simulink library "lib_lowphy"  (R2023b)
settings: Solver=VariableStepAuto  StartTime=0.0  StopTime=10.0  RelTol=1e-3
undefined symbols (not defined in the file or in its folder): AdvDSPBChannelOutDisplay, AdvDSPBDMemDisplay, AdvDSPBInDisplay, AdvDSPBOutDisplay, dpoly, dspba, dspba_ChannelInVis, dspba_ChannelOutVis, dspba_internal_get_channel_ports, evalAionMaskParam, fft_tb_in, ifft_tb_in, latency, latencyCorrection, max_FFTStages, max_NSubcarriers, primtype, UseDontCare, value
libraries: DSPBAPrim x637, DSPBAControl x55, $bdroot x16, DSPBAModelBus x12, DSPBAUtilities x6, DSPBABase x5, DSPBAWaveformSynth x4, DspbAdvFftLibrary x3, DSPBAVectorUtil x2, DspbAdvVfftPrefix x1
(part 7 of 9)

== system lib_lowphy/iFFT_B2S/B2S/B2S_Inst/CB/Rdaddr_gen1 ==
  sampleaddr_reg : Inport
  cpin : Inport  Port=2
  rba : Inport  Port=3
  fftsize : Inport  Port=4
  Lut4 : DSPBAPrim/Lut  primtype=lut  nInputs=1  nOutputs=1  omode=Specify via dialog  otype=fixdt(0,2,0)  scale=0  rndmethod=Unbiased  factor=1  satmethod=Symmetric  shift_vec=[0 1 2 -1]  value=[0 zeros(1,8) 0 1 2 3 0]  inPortNames=[' '; ' ';]  outPortNames=[' ']  dspbaimage=dspba_prim.svg  text=fprintf('LUT');  style=Optimised  visibilities=8 + 1024  floatPrecision=float32_m23  version=20211007
  Mux : DSPBAPrim/Mux  primtype=mux  nInputs=evalAionMaskParam(gcb,'value',1)+1  nOutputs=1  omode=Inherit via internal rule  otype=sfix(16)  scale=2^-15  rndmethod=Unbiased  factor=1  satmethod=Symmetric  shift_vec=[0 1 2 -1]  value=4  inPortNames=['s '; 'd0'; 'd1'; 'd2'; 'd3'; 'd4'; 'd5'; 'd6'; 'd7'; 'd8'; 'd9';]  outPortNames=[' ']  dspbaimage=dspba_prim_tall.svg  text=fprintf('%s', primtype);  style=Optimised  visibilities=1032  version=20211007
  Mux1 : DSPBAPrim/Mux  primtype=mux  nInputs=evalAionMaskParam(gcb,'value',1)+1  nOutputs=1  omode=Inherit via internal rule  otype=sfix(16)  scale=2^-15  rndmethod=Unbiased  factor=1  satmethod=Symmetric  shift_vec=[0 1 2 -1]  value=4  inPortNames=['s '; 'd0'; 'd1'; 'd2'; 'd3'; 'd4'; 'd5'; 'd6'; 'd7'; 'd8'; 'd9';]  outPortNames=[' ']  dspbaimage=dspba_prim_tall.svg  text=fprintf('%s', primtype);  style=Optimised  visibilities=1032  version=20211007
  rd_addr_1024 : Subsystem
  rd_addr_2048 : Subsystem
  rd_addr_512 : Subsystem
  rd_addr_gen_4096 : Subsystem
  AntNo : Outport
  rdaddr1 : Outport  Port=2
  rbaout : Outport  Port=3
  wires:
  cpin/1 -> rd_addr_2048/2(cpin), rd_addr_512/2(cpin), rd_addr_1024/2(cpin), rd_addr_gen_4096/2(cpin)
  sampleaddr_reg/1 -> rd_addr_512/1(sampleaddr_reg), rd_addr_1024/1(sampleaddr_reg), rd_addr_2048/1(sampleaddr_reg), rd_addr_gen_4096/1(sampleaddr_reg)
  rba/1 -> rbaout/1
  fftsize/1 -> Lut4/1
  Mux/1 -> AntNo/1
  Mux1/1 -> rdaddr1/1
  Lut4/1 -> Mux1/1, Mux/1
  rd_addr_512/1(AntNo) -> Mux/2
  rd_addr_1024/1(AntNo) -> Mux/3
  rd_addr_2048/1(AntNo) -> Mux/4
  rd_addr_gen_4096/1(AntNo) -> Mux/5
  rd_addr_gen_4096/2(rdaddr1) -> Mux1/5
  rd_addr_2048/2(rdaddr1) -> Mux1/4
  rd_addr_1024/2(rdaddr1) -> Mux1/3
  rd_addr_512/2(rdaddr1) -> Mux1/2

== system lib_lowphy/iFFT_B2S/B2S/B2S_Inst/CB/SampleReggen ==
  note: Look Ahead Go Pulse Gen
  note: Min_delay and fixed
  note: rba generation
  note: Min_delay 8 and fixed as 1+6+1
  note: latch the cp ot & sample size before process
  CPlen : Inport
  FFTSize : Inport  Port=2
  wba : Inport  Port=3
  Symno : Inport  Port=4
  Constant : Constant  OutDataTypeStr=boolean
  Counter_go_enable_sig : Subsystem
  EndCounterSignals : Subsystem
  LastSig_delay : DSPBAPrim/SampleDelay  primtype=sampdelay  nInputs=1  nOutputs=1  omode=boolean  otype=sfix(16)  scale=2^-15  rndmethod=Unbiased  factor=1  satmethod=Symmetric  shift_vec=[0 1 2 -1]  floatPrecision=float32_m23  value=14  inPortNames=[' '; ' ';]  outPortNames=[' ']  dspbaimage=dspba_prim.svg  text=dpoly(1, eye(1,value+1), 'z')  style=Optimised  visibilities=8 + 1024 + 2^17 + 2^18  flexible=off  slackgroup=0  augmented=1  version=20211007  advOptions=[]
  Mux : DSPBAPrim/Mux  primtype=mux  nInputs=evalAionMaskParam(gcb,'value',1)+1  nOutputs=1  omode=Inherit via internal rule  otype=sfix(16)  scale=2^-15  rndmethod=Unbiased  factor=1  satmethod=Symmetric  shift_vec=[0 1 2 -1]  value=2  inPortNames=['s '; 'd0'; 'd1'; 'd2'; 'd3'; 'd4'; 'd5'; 'd6'; 'd7'; 'd8'; 'd9';]  outPortNames=[' ']  dspbaimage=dspba_prim_tall.svg  text=fprintf('%s', primtype);  style=Optimised  visibilities=1032  version=20211007
  Not : DSPBAPrim/Not  primtype=not  nInputs=1  nOutputs=1  omode=Inherit via internal rule  otype=sfix(16)  scale=2^-15  rndmethod=Unbiased  factor=1  satmethod=Symmetric  shift_vec=[0 1 2 -1]  value=0  inPortNames=[' '; ' ';]  outPortNames=[' ']  dspbaimage=dspba_prim.svg  text=fprintf('~');  style=Optimised  visibilities=8  version=20211007
  SampleregMaxval_Calc2 : Subsystem
  Valid2 : DSPBAPrim/SampleDelay  primtype=sampdelay  nInputs=1  nOutputs=1  omode=boolean  otype=sfix(16)  scale=2^-15  rndmethod=Unbiased  factor=1  satmethod=Symmetric  shift_vec=[0 1 2 -1]  floatPrecision=float32_m23  value=1  inPortNames=[' '; ' ';]  outPortNames=[' ']  dspbaimage=dspba_prim.svg  text=dpoly(1, eye(1,value+1), 'z')  style=Optimised  visibilities=8 + 1024 + 2^17 + 2^18  flexible=off  slackgroup=0  augmented=7  version=20211007  advOptions=[]
  WriteOnlyLoop : DSPBAPrim/Loop  primtype=loop  nInputs=3  nOutputs=4  omode=Inherit via internal rule  otype=sfix(16)  scale=2^-15  rndmethod=Unbiased  factor=1  satmethod=Symmetric  shift_vec=[0 1 2 -1]  value=[zeros(16, 1)]  inPortNames=['g'; 'c'; 'e']  outPortNames=['v'; 'q'; 'f'; 'l']  dspbaimage=dspba_prim_tall.svg  text=fprintf('loop');  style=Optimised  visibilities=0  version=20211007
  _sample_maxlatch_0L : DSPBAControl/latch_0L
  _sample_maxlatch_0L1 : DSPBAControl/latch_0L
  rbaValid : DSPBAPrim/SampleDelay  primtype=sampdelay  nInputs=1  nOutputs=1  omode=boolean  otype=sfix(16)  scale=2^-15  rndmethod=Unbiased  factor=1  satmethod=Symmetric  shift_vec=[0 1 2 -1]  floatPrecision=float32_m23  value=1  inPortNames=[' '; ' ';]  outPortNames=[' ']  dspbaimage=dspba_prim.svg  text=dpoly(1, eye(1,value+1), 'z')  style=Optimised  visibilities=8 + 1024 + 2^17 + 2^18  flexible=off  slackgroup=0  augmented=1  version=20211007  advOptions=[]
  rbaValid1 : DSPBAPrim/SampleDelay  primtype=sampdelay  nInputs=1  nOutputs=1  omode=boolean  otype=sfix(16)  scale=2^-15  rndmethod=Unbiased  factor=1  satmethod=Symmetric  shift_vec=[0 1 2 -1]  floatPrecision=float32_m23  value=6+7  inPortNames=[' '; ' ';]  outPortNames=[' ']  dspbaimage=dspba_prim.svg  text=dpoly(1, eye(1,value+1), 'z')  style=Optimised  visibilities=8 + 1024 + 2^17 + 2^18  flexible=off  slackgroup=0  augmented=1  version=20211007  advOptions=[]
  validout : Outport
  samplecntreg_final : Outport  Port=2
  first : Outport  Port=3
  last : Outport  Port=4
  running : Outport  Port=5
  rba_final : Outport  Port=6
  cp_out : Outport  Port=7
  wires:
  WriteOnlyLoop/1 -> EndCounterSignals/3(validin), validout/1, Counter_go_enable_sig/2(running)
  WriteOnlyLoop/2 -> samplecntreg_final/1, EndCounterSignals/1(Count_in)
  WriteOnlyLoop/3 -> last/1, first/1
  WriteOnlyLoop/4 -> running/1
  Constant/1 -> WriteOnlyLoop/3
  wba/1 -> Counter_go_enable_sig/1(wba)  "wba"
  CPlen/1 -> SampleregMaxval_Calc2/3(cplen)
  [LastCountMinFifteen] -> Mux/1
  Mux/1 -> Valid2/1
  Valid2/1 -> Mux/2, Not/1, rbaValid1/1
  Not/1 -> Mux/3
  _sample_maxlatch_0L/1 -> WriteOnlyLoop/2, EndCounterSignals/2(Count_max)  "log_loopCval"
  EndCounterSignals/1(Last_Minus_two) -> [LastCountMintwo]
  EndCounterSignals/2(Last_Minus_one) -> [LastCountMinone]
  EndCounterSignals/3(Last_Minus_eight) -> [LastCountMineight]
  EndCounterSignals/4(Last_Minus_fifteen) -> [LastCountMinFifteen]
  Counter_go_enable_sig/1(Go) -> WriteOnlyLoop/1, _sample_maxlatch_0L/1, _sample_maxlatch_0L1/1  "log_go_sig"
  LastSig_delay/1 -> Counter_go_enable_sig/4(Counterend)
  [LastCountMinFifteen] -> LastSig_delay/1
  [rba_Lookahead] -> Counter_go_enable_sig/3(rba)
  rbaValid/1 -> [rba], rba_final/1
  rbaValid1/1 -> [rba_Lookahead], rbaValid/1
  SampleregMaxval_Calc2/1(SampleregMaxval) -> _sample_maxlatch_0L/2  "log_sampleregmaxval"
  FFTSize/1 -> SampleregMaxval_Calc2/1(FFTSize)
  Symno/1 -> SampleregMaxval_Calc2/2(sym_num)
  SampleregMaxval_Calc2/2(cp_out) -> _sample_maxlatch_0L1/2
  _sample_maxlatch_0L1/1 -> cp_out/1

== system lib_lowphy/iFFT_B2S/B2S/B2S_Inst/CB/Wr_addr_Gen2 ==
  en_in : Inport
  fft_size : Inport  Port=2
  nprb : Inport  Port=3
  Delay_rd_go_pulse : $bdroot/iFFT_B2S/B2S/B2S_Inst/CB/Wr_addr_Gen2/Delay_rd_go  Commented=on  SystemSampleTime=-1  SSRTWFcnClass=[]  VariantActivationTime=update diagram  Latency=0  AutoFrameSizeCalculation=off
  Terminator : Terminator
  Wr_addr_Gen2 : Subsystem
  wba_flag : Outport
  Antenna_no : Outport  Port=2
  Complete_wr_addr : Outport  Port=3
  wires:
  en_in/1 -> Wr_addr_Gen2/1(en_in)
  Wr_addr_Gen2/1(wba_flag) -> wba_flag/1  "wba_flag"
  Wr_addr_Gen2/2(Antenna_no) -> Antenna_no/1  "Wr_Antenna_no"
  Wr_addr_Gen2/3(Complete_wr_addr) -> Complete_wr_addr/1  "Wr_ptr"
  fft_size/1 -> Wr_addr_Gen2/2(fft_size)
  nprb/1 -> Terminator/1

== system lib_lowphy/iFFT_B2S/B2S/B2S_Inst/CB/edgedetector ==
  signal : Inport
  SampleDelay : DSPBAPrim/SampleDelay  primtype=sampdelay  nInputs=1  nOutputs=1  omode=Inherit via internal rule  otype=sfix(16)  scale=2^-15  rndmethod=Unbiased  factor=1  satmethod=Symmetric  shift_vec=[0 1 2 -1]  floatPrecision=float32_m23  value=1  inPortNames=[' '; ' ';]  outPortNames=[' ']  dspbaimage=dspba_prim.svg  text=dpoly(1, eye(1,value+1), 'z')  style=Optimised  visibilities=8 + 1024 + 2^17 + 2^18  flexible=off  slackgroup=0  augmented=0  version=20211007  advOptions=[]
  Xor : DSPBAPrim/Xor  primtype=xor  nInputs=2  nOutputs=1  omode=Inherit via internal rule  otype=sfix(16)  scale=2^-15  rndmethod=Unbiased  factor=1  satmethod=Symmetric  shift_vec=[0 1 2 -1]  value=0  inPortNames=[' '; ' '; ' '; ' '; ' '; ' '; ' '; ' '; ' '; ' '; ' '; ' '; ' '; ' '; ' '; ' '; ]  outPortNames=[' ']  dspbaimage=dspba_prim.svg  text=fprintf('^');  style=Optimised  visibilities=8+2  version=20211007
  edge : Outport
  wires:
  SampleDelay/1 -> Xor/1
  signal/1 -> Xor/2, SampleDelay/1
  Xor/1 -> edge/1

== system lib_lowphy/iFFT_B2S/B2S/B2S_Inst/MemandMux/Subsystem ==
  dv : Inport
  AntennaNo : Inport  Port=2
  AntennaCurId : Inport  Port=3
  data_in : Inport  Port=4
  Wraddr : Inport  Port=5
  rdaddr : Inport  Port=6
  CmpEQ : DSPBAPrim/CmpEQ  primtype=cmpeq  nInputs=2  nOutputs=1  omode=boolean  otype=sfix(16)  scale=2^-15  rndmethod=Unbiased  factor=1  satmethod=Symmetric  shift_vec=[0 1 2 -1]  value=0  inPortNames=[' '; ' ';]  outPortNames=[' ']  dspbaimage=dspba_prim.svg  text=fprintf('==');  style=Optimised  visibilities=0  advOptions=[]  version=20211007
  MemArray : DSPBAPrim/DualMem  primtype=dualmem  nInputs=4  nOutputs=2  omode=Inherit via internal rule  otype=sfix(16)  scale=2^-15  rndmethod=Unbiased  factor=1  satmethod=Symmetric  shift_vec=[0 1 2 -1]  value=[zeros(2^(max_FFTStages+1), 1)]  inPortNames=['d1'; 'a1'; 'w1'; 'a2']  outPortNames=['q1'; 'q2']  dspbaimage=dspba_prim_tall.svg  text=fprintf('dmem%s',AdvDSPBDMemDisplay(UseDontCare));  style=Optimised  visibilities=8 + 1024 + 2^17 + 2^18  UseDontCare=on  TwinWritePorts=off  init=on  ProvideReadAccess=off  version=20211007
  Terminator : Terminator
  We_mem1 : DSPBAPrim/And  primtype=and  nInputs=2  nOutputs=1  omode=Inherit via internal rule  otype=sfix(16)  scale=2^-15  rndmethod=Unbiased  factor=1  satmethod=Symmetric  shift_vec=[0 1 2 -1]  value=0  inPortNames=[' '; ' '; ' '; ' '; ' '; ' '; ' '; ' '; ' '; ' '; ' '; ' '; ' '; ' '; ' '; ' '; ]  outPortNames=[' ']  dspbaimage=dspba_prim.svg  text=fprintf('&');  style=Optimised  visibilities=8+2  version=20211007
  rddata : Outport
  wires:
  MemArray/2 -> rddata/1
  data_in/1 -> MemArray/1  "mod_mem_wr_data_in"
  dv/1 -> We_mem1/2
  We_mem1/1 -> MemArray/3  "mod_mem_wr_en_in"
  MemArray/1 -> Terminator/1
  AntennaCurId/1 -> CmpEQ/1
  AntennaNo/1 -> CmpEQ/2
  CmpEQ/1 -> We_mem1/1
  Wraddr/1 -> MemArray/2  "mod_mem_wr_addr_in"
  rdaddr/1 -> MemArray/4

== system lib_lowphy/iFFT_B2S/B2S/B2S_Inst/MemandMux/Subsystem1 ==
  dv : Inport
  AntennaNo : Inport  Port=2
  AntennaCurId : Inport  Port=3
  data_in : Inport  Port=4
  Wraddr : Inport  Port=5
  rdaddr : Inport  Port=6
  CmpEQ : DSPBAPrim/CmpEQ  primtype=cmpeq  nInputs=2  nOutputs=1  omode=boolean  otype=sfix(16)  scale=2^-15  rndmethod=Unbiased  factor=1  satmethod=Symmetric  shift_vec=[0 1 2 -1]  value=0  inPortNames=[' '; ' ';]  outPortNames=[' ']  dspbaimage=dspba_prim.svg  text=fprintf('==');  style=Optimised  visibilities=0  advOptions=[]  version=20211007
  MemArray : DSPBAPrim/DualMem  primtype=dualmem  nInputs=4  nOutputs=2  omode=Inherit via internal rule  otype=sfix(16)  scale=2^-15  rndmethod=Unbiased  factor=1  satmethod=Symmetric  shift_vec=[0 1 2 -1]  value=[zeros(2^(max_FFTStages+1), 1)]  inPortNames=['d1'; 'a1'; 'w1'; 'a2']  outPortNames=['q1'; 'q2']  dspbaimage=dspba_prim_tall.svg  text=fprintf('dmem%s',AdvDSPBDMemDisplay(UseDontCare));  style=Optimised  visibilities=8 + 1024 + 2^17 + 2^18  UseDontCare=on  TwinWritePorts=off  init=on  ProvideReadAccess=off  version=20211007
  Terminator : Terminator
  We_mem3 : DSPBAPrim/And  primtype=and  nInputs=2  nOutputs=1  omode=Inherit via internal rule  otype=sfix(16)  scale=2^-15  rndmethod=Unbiased  factor=1  satmethod=Symmetric  shift_vec=[0 1 2 -1]  value=0  inPortNames=[' '; ' '; ' '; ' '; ' '; ' '; ' '; ' '; ' '; ' '; ' '; ' '; ' '; ' '; ' '; ' '; ]  outPortNames=[' ']  dspbaimage=dspba_prim.svg  text=fprintf('&');  style=Optimised  visibilities=8+2  version=20211007
  rddata : Outport
  wires:
  MemArray/2 -> rddata/1
  data_in/1 -> MemArray/1
  dv/1 -> We_mem3/2
  We_mem3/1 -> MemArray/3
  MemArray/1 -> Terminator/1
  AntennaCurId/1 -> CmpEQ/1
  AntennaNo/1 -> CmpEQ/2
  CmpEQ/1 -> We_mem3/1
  Wraddr/1 -> MemArray/2
  rdaddr/1 -> MemArray/4

== system lib_lowphy/iFFT_B2S/B2S/B2S_Inst/MemandMux/Subsystem2 ==
  dv : Inport
  AntennaNo : Inport  Port=2
  AntennaCurId : Inport  Port=3
  data_in : Inport  Port=4
  Wraddr : Inport  Port=5
  rdaddr : Inport  Port=6
  CmpEQ : DSPBAPrim/CmpEQ  primtype=cmpeq  nInputs=2  nOutputs=1  omode=boolean  otype=sfix(16)  scale=2^-15  rndmethod=Unbiased  factor=1  satmethod=Symmetric  shift_vec=[0 1 2 -1]  value=0  inPortNames=[' '; ' ';]  outPortNames=[' ']  dspbaimage=dspba_prim.svg  text=fprintf('==');  style=Optimised  visibilities=0  advOptions=[]  version=20211007
  MemArray : DSPBAPrim/DualMem  primtype=dualmem  nInputs=4  nOutputs=2  omode=Inherit via internal rule  otype=sfix(16)  scale=2^-15  rndmethod=Unbiased  factor=1  satmethod=Symmetric  shift_vec=[0 1 2 -1]  value=[zeros(2^(max_FFTStages+1), 1)]  inPortNames=['d1'; 'a1'; 'w1'; 'a2']  outPortNames=['q1'; 'q2']  dspbaimage=dspba_prim_tall.svg  text=fprintf('dmem%s',AdvDSPBDMemDisplay(UseDontCare));  style=Optimised  visibilities=8 + 1024 + 2^17 + 2^18  UseDontCare=on  TwinWritePorts=off  init=on  ProvideReadAccess=off  version=20211007
  Terminator : Terminator
  We_mem2 : DSPBAPrim/And  primtype=and  nInputs=2  nOutputs=1  omode=Inherit via internal rule  otype=sfix(16)  scale=2^-15  rndmethod=Unbiased  factor=1  satmethod=Symmetric  shift_vec=[0 1 2 -1]  value=0  inPortNames=[' '; ' '; ' '; ' '; ' '; ' '; ' '; ' '; ' '; ' '; ' '; ' '; ' '; ' '; ' '; ' '; ]  outPortNames=[' ']  dspbaimage=dspba_prim.svg  text=fprintf('&');  style=Optimised  visibilities=8+2  version=20211007
  rddata : Outport
  wires:
  MemArray/2 -> rddata/1
  data_in/1 -> MemArray/1
  dv/1 -> We_mem2/2
  We_mem2/1 -> MemArray/3
  MemArray/1 -> Terminator/1
  AntennaCurId/1 -> CmpEQ/1
  AntennaNo/1 -> CmpEQ/2
  CmpEQ/1 -> We_mem2/1
  Wraddr/1 -> MemArray/2
  rdaddr/1 -> MemArray/4

== system lib_lowphy/iFFT_B2S/B2S/B2S_Inst/MemandMux/Subsystem3 ==
  dv : Inport
  AntennaNo : Inport  Port=2
  AntennaCurId : Inport  Port=3
  data_in : Inport  Port=4
  Wraddr : Inport  Port=5
  rdaddr : Inport  Port=6
  CmpEQ : DSPBAPrim/CmpEQ  primtype=cmpeq  nInputs=2  nOutputs=1  omode=boolean  otype=sfix(16)  scale=2^-15  rndmethod=Unbiased  factor=1  satmethod=Symmetric  shift_vec=[0 1 2 -1]  value=0  inPortNames=[' '; ' ';]  outPortNames=[' ']  dspbaimage=dspba_prim.svg  text=fprintf('==');  style=Optimised  visibilities=0  advOptions=[]  version=20211007
  MemArray : DSPBAPrim/DualMem  primtype=dualmem  nInputs=4  nOutputs=2  omode=Inherit via internal rule  otype=sfix(16)  scale=2^-15  rndmethod=Unbiased  factor=1  satmethod=Symmetric  shift_vec=[0 1 2 -1]  value=[zeros(2^(max_FFTStages+1), 1)]  inPortNames=['d1'; 'a1'; 'w1'; 'a2']  outPortNames=['q1'; 'q2']  dspbaimage=dspba_prim_tall.svg  text=fprintf('dmem%s',AdvDSPBDMemDisplay(UseDontCare));  style=Optimised  visibilities=8 + 1024 + 2^17 + 2^18  UseDontCare=on  TwinWritePorts=off  init=on  ProvideReadAccess=off  version=20211007
  Terminator : Terminator
  We_mem4 : DSPBAPrim/And  primtype=and  nInputs=2  nOutputs=1  omode=Inherit via internal rule  otype=sfix(16)  scale=2^-15  rndmethod=Unbiased  factor=1  satmethod=Symmetric  shift_vec=[0 1 2 -1]  value=0  inPortNames=[' '; ' '; ' '; ' '; ' '; ' '; ' '; ' '; ' '; ' '; ' '; ' '; ' '; ' '; ' '; ' '; ]  outPortNames=[' ']  dspbaimage=dspba_prim.svg  text=fprintf('&');  style=Optimised  visibilities=8+2  version=20211007
  rddata : Outport
  wires:
  MemArray/2 -> rddata/1
  data_in/1 -> MemArray/1
  dv/1 -> We_mem4/2
  We_mem4/1 -> MemArray/3
  MemArray/1 -> Terminator/1
  AntennaCurId/1 -> CmpEQ/1
  AntennaNo/1 -> CmpEQ/2
  CmpEQ/1 -> We_mem4/1
  Wraddr/1 -> MemArray/2
  rdaddr/1 -> MemArray/4

== system lib_lowphy/iFFT_B2S/IFFT/VIFFT/BRandSCMap/Subsystem ==
  qv : Inport
  v : Inport  Port=2
  d : Inport  Port=3
  FIFO : DSPBAPrim/FIFO  primtype=fifo  nInputs=3  nOutputs=4  omode=Inherit via internal rule  otype=sfix(16)  scale=2^-15  rndmethod=Unbiased  factor=1  satmethod=Symmetric  shift_vec=[0 1 2 -1]  value=[16 16 16]  inPortNames=['w'; 'd'; 'r'; 'f']  outPortNames=['v'; 'q'; 't'; 'f']  dspbaimage=dspba_prim_tall.svg  text=fprintf('fifo');  style=Optimised  visibilities=263168  version=20211007  user_sclr=off
  RISING_EDGE1 : Subsystem
  RISING_EDGE3 : Subsystem
  Terminator1 : Terminator
  Terminator2 : Terminator
  Terminator3 : Terminator
  latch_0L3 : DSPBAControl/latch_0L
  q : Outport
  wires:
  FIFO/2 -> latch_0L3/2
  RISING_EDGE3/1(q) -> latch_0L3/1, FIFO/3
  FIFO/3 -> Terminator2/1
  latch_0L3/1 -> q/1
  d/1 -> FIFO/2
  FIFO/4 -> Terminator3/1
  v/1 -> RISING_EDGE1/1(d)
  qv/1 -> RISING_EDGE3/1(d)
  FIFO/1 -> Terminator1/1
  RISING_EDGE1/1(q) -> FIFO/1

== system lib_lowphy/iFFT_B2S/IFFT/VIFFT/BRandSCMap/Subsystem1 ==
  qv : Inport
  v : Inport  Port=2
  d : Inport  Port=3
  FIFO : DSPBAPrim/FIFO  primtype=fifo  nInputs=3  nOutputs=4  omode=Inherit via internal rule  otype=sfix(16)  scale=2^-15  rndmethod=Unbiased  factor=1  satmethod=Symmetric  shift_vec=[0 1 2 -1]  value=[16 16 16]  inPortNames=['w'; 'd'; 'r'; 'f']  outPortNames=['v'; 'q'; 't'; 'f']  dspbaimage=dspba_prim_tall.svg  text=fprintf('fifo');  style=Optimised  visibilities=263168  version=20211007  user_sclr=off
  RISING_EDGE1 : Subsystem
  RISING_EDGE3 : Subsystem
  Terminator1 : Terminator
  Terminator2 : Terminator
  Terminator3 : Terminator
  latch_0L3 : DSPBAControl/latch_0L
  q : Outport
  wires:
  FIFO/1 -> Terminator1/1
  qv/1 -> RISING_EDGE3/1(d)
  v/1 -> RISING_EDGE1/1(d)
  FIFO/4 -> Terminator3/1
  d/1 -> FIFO/2
  latch_0L3/1 -> q/1
  FIFO/3 -> Terminator2/1
  RISING_EDGE3/1(q) -> FIFO/3, latch_0L3/1
  FIFO/2 -> latch_0L3/2
  RISING_EDGE1/1(q) -> FIFO/1

== system lib_lowphy/iFFT_B2S/IFFT/VIFFT/BRandSCMap/Subsystem2 ==
  qv : Inport
  v : Inport  Port=2
  d : Inport  Port=3
  FIFO : DSPBAPrim/FIFO  primtype=fifo  nInputs=3  nOutputs=4  omode=Inherit via internal rule  otype=sfix(16)  scale=2^-15  rndmethod=Unbiased  factor=1  satmethod=Symmetric  shift_vec=[0 1 2 -1]  value=[16 16 16]  inPortNames=['w'; 'd'; 'r'; 'f']  outPortNames=['v'; 'q'; 't'; 'f']  dspbaimage=dspba_prim_tall.svg  text=fprintf('fifo');  style=Optimised  visibilities=263168  version=20211007  user_sclr=off
  RISING_EDGE1 : Subsystem
  RISING_EDGE3 : Subsystem
  Terminator1 : Terminator
  Terminator2 : Terminator
  Terminator3 : Terminator
  latch_0L3 : DSPBAControl/latch_0L
  q : Outport
  wires:
  FIFO/2 -> latch_0L3/2
  RISING_EDGE3/1(q) -> latch_0L3/1, FIFO/3
  FIFO/3 -> Terminator2/1
  latch_0L3/1 -> q/1
  d/1 -> FIFO/2
  FIFO/4 -> Terminator3/1
  v/1 -> RISING_EDGE1/1(d)
  qv/1 -> RISING_EDGE3/1(d)
  FIFO/1 -> Terminator1/1
  RISING_EDGE1/1(q) -> FIFO/1

== system lib_lowphy/iFFT_B2S/IFFT/VIFFT/BRandSCMap/Subsystem3 ==
  qv : Inport
  v : Inport  Port=2
  d : Inport  Port=3
  FIFO : DSPBAPrim/FIFO  primtype=fifo  nInputs=3  nOutputs=4  omode=Inherit via internal rule  otype=sfix(16)  scale=2^-15  rndmethod=Unbiased  factor=1  satmethod=Symmetric  shift_vec=[0 1 2 -1]  value=[16 16 16]  inPortNames=['w'; 'd'; 'r'; 'f']  outPortNames=['v'; 'q'; 't'; 'f']  dspbaimage=dspba_prim_tall.svg  text=fprintf('fifo');  style=Optimised  visibilities=263168  version=20211007  user_sclr=off
  RISING_EDGE1 : Subsystem
  RISING_EDGE3 : Subsystem
  Terminator1 : Terminator
  Terminator2 : Terminator
  Terminator3 : Terminator
  latch_0L3 : DSPBAControl/latch_0L
  q : Outport
  wires:
  FIFO/2 -> latch_0L3/2
  RISING_EDGE3/1(q) -> latch_0L3/1, FIFO/3
  FIFO/3 -> Terminator2/1
  latch_0L3/1 -> q/1
  d/1 -> FIFO/2
  FIFO/4 -> Terminator3/1
  v/1 -> RISING_EDGE1/1(d)
  qv/1 -> RISING_EDGE3/1(d)
  FIFO/1 -> Terminator1/1
  RISING_EDGE1/1(q) -> FIFO/1

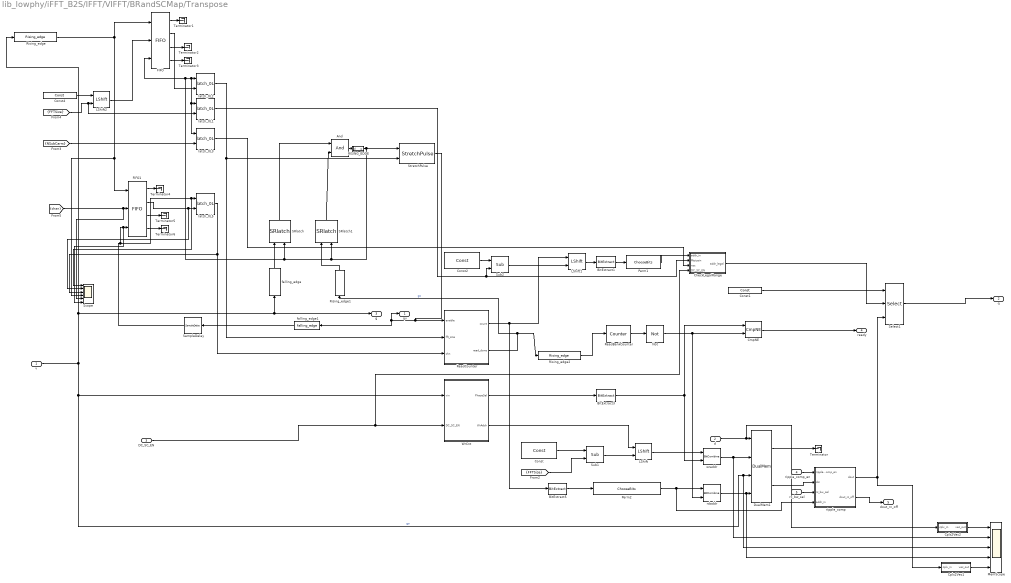
== system lib_lowphy/iFFT_B2S/IFFT/VIFFT/BRandSCMap/Transpose ==
  v : Inport
  d : Inport  Port=2
  DC_SC_EN : Inport  Port=3
  ripple_comp_en : Inport  Port=4
  rc_bw_sel : Inport  Port=5
  And : DSPBAPrim/And  primtype=and  nInputs=2  nOutputs=1  omode=Inherit via internal rule  otype=sfix(16)  scale=2^-15  rndmethod=Unbiased  factor=1  satmethod=Symmetric  shift_vec=[0 1 2 -1]  value=0  inPortNames=[' '; ' '; ' '; ' '; ' '; ' '; ' '; ' '; ' '; ' '; ' '; ' '; ' '; ' '; ' '; ' '; ]  outPortNames=[' ']  dspbaimage=dspba_prim.svg  text=fprintf('&');  style=Optimised  visibilities=8+2  version=20211007
  BitExtract1 : DSPBAPrim/BitExtract  primtype=bitextract  nInputs=1  nOutputs=1  omode=Specify via dialog  otype=ufix(max_FFTStages)  scale=1  rndmethod=Unbiased  factor=1  satmethod=Symmetric  shift_vec=[0 1 2 -1]  value=0  inPortNames=[' '; ' ';]  outPortNames=[' ']  dspbaimage=dspba_prim.svg  text=fprintf('..%d', value);  style=Optimised  visibilities=8 + 1024  version=20211007
  BitExtract3 : DSPBAPrim/BitExtract  primtype=bitextract  nInputs=1  nOutputs=1  omode=boolean  otype=ufix(N)  scale=1  rndmethod=Unbiased  factor=1  satmethod=Symmetric  shift_vec=[0 1 2 -1]  value=0  inPortNames=[' '; ' ';]  outPortNames=[' ']  dspbaimage=dspba_prim.svg  text=fprintf('..%d', value);  style=Optimised  visibilities=8 + 1024  version=20211007
  BitExtract5 : DSPBAPrim/BitExtract  primtype=bitextract  nInputs=1  nOutputs=1  omode=Specify via dialog  otype=ufix(max_FFTStages)  scale=1  rndmethod=Unbiased  factor=1  satmethod=Symmetric  shift_vec=[0 1 2 -1]  value=0  inPortNames=[' '; ' ';]  outPortNames=[' ']  dspbaimage=dspba_prim.svg  text=fprintf('..%d', value);  style=Optimised  visibilities=8 + 1024  version=20211007
  CheckLegalRange : Subsystem
  CmpNE : DSPBAPrim/CmpNE  primtype=cmpne  nInputs=2  nOutputs=1  omode=boolean  otype=sfix(16)  scale=2^-15  rndmethod=Unbiased  factor=1  satmethod=Symmetric  shift_vec=[0 1 2 -1]  value=0  inPortNames=[' '; ' ';]  outPortNames=[' ']  dspbaimage=dspba_prim.svg  text=fprintf('~=');  style=Optimised  visibilities=0  advOptions=[]  version=20211007
  Const : DSPBAPrim/Const  primtype=const  nInputs=0  nOutputs=1  omode=Specify via dialog  otype=ufix(ceil(log2(max_FFTStages)))  scale=1  rndmethod=Unbiased  factor=1  satmethod=Symmetric  shift_vec=[0 1 2 -1]  value=max_FFTStages  inPortNames=['+'; '+';]  outPortNames=[' ']  dspbaimage=dspba_prim.svg  text=fprintf('%s', num2str(value));  style=Optimised  visibilities=8 + 1024  floatPrecision=float32_m23  warnSaturation=on  version=20211007  SampleTime=inf
  Const1 : DSPBAPrim/Const  primtype=const  nInputs=0  nOutputs=1  omode=Inherit via internal rule  otype=sfix(16)  scale=2^-15  rndmethod=Unbiased  factor=1  satmethod=Symmetric  shift_vec=[0 1 2 -1]  value=0  inPortNames=['+'; '+';]  outPortNames=[' ']  dspbaimage=dspba_prim.svg  text=fprintf('%s', num2str(value));  style=Optimised  visibilities=8 + 1024  floatPrecision=float32_m23  warnSaturation=on  version=20211007  SampleTime=inf
  Const2 : DSPBAPrim/Const  primtype=const  nInputs=0  nOutputs=1  omode=Specify via dialog  otype=ufix(ceil(log2(max_FFTStages)))  scale=1  rndmethod=Unbiased  factor=1  satmethod=Symmetric  shift_vec=[0 1 2 -1]  value=max_FFTStages  inPortNames=['+'; '+';]  outPortNames=[' ']  dspbaimage=dspba_prim.svg  text=fprintf('%s', num2str(value));  style=Optimised  visibilities=8 + 1024  floatPrecision=float32_m23  warnSaturation=on  version=20211007  SampleTime=inf
  Const4 : DSPBAPrim/Const  primtype=const  nInputs=0  nOutputs=1  omode=Inherit via internal rule  otype=sfix(16)  scale=2^-15  rndmethod=Unbiased  factor=1  satmethod=Symmetric  shift_vec=[0 1 2 -1]  value=1  inPortNames=['+'; '+';]  outPortNames=[' ']  dspbaimage=dspba_prim.svg  text=fprintf('%s', num2str(value));  style=Optimised  visibilities=8 + 1024  floatPrecision=float32_m23  warnSaturation=on  version=20211007  SampleTime=inf
  Cplx2Vec1 : Subsystem
  Cplx2Vec2 : Subsystem
  DualMem1 : DSPBAPrim/DualMem  primtype=dualmem  nInputs=4  nOutputs=2  omode=Inherit via internal rule  otype=sfix(16)  scale=2^-15  rndmethod=Unbiased  factor=1  satmethod=Symmetric  shift_vec=[0 1 2 -1]  value=[zeros(2^(max_FFTStages+1), 1)]  inPortNames=['d1'; 'a1'; 'w1'; 'a2']  outPortNames=['q1'; 'q2']  dspbaimage=dspba_prim_tall.svg  text=fprintf('dmem');  style=Optimised  visibilities=8 + 1024  UseDontCare=on  TwinWritePorts=off  init=on  ProvideReadAccess=off  version=20211007
  FIFO : DSPBAPrim/FIFO  primtype=fifo  nInputs=3  nOutputs=4  omode=Inherit via internal rule  otype=sfix(16)  scale=2^-15  rndmethod=Unbiased  factor=1  satmethod=Symmetric  shift_vec=[0 1 2 -1]  value=[16 16 16]  inPortNames=['w'; 'd'; 'r'; 'f']  outPortNames=['v'; 'q'; 't'; 'f']  dspbaimage=dspba_prim_tall.svg  text=fprintf('fifo');  style=Optimised  visibilities=263168  version=20211007  user_sclr=off
  FIFO1 : DSPBAPrim/FIFO  primtype=fifo  nInputs=3  nOutputs=4  omode=Inherit via internal rule  otype=sfix(16)  scale=2^-15  rndmethod=Unbiased  factor=1  satmethod=Symmetric  shift_vec=[0 1 2 -1]  value=[16 16 16]  inPortNames=['w'; 'd'; 'r'; 'f']  outPortNames=['v'; 'q'; 't'; 'f']  dspbaimage=dspba_prim_tall.svg  text=fprintf('fifo');  style=Optimised  visibilities=263168  version=20211007  user_sclr=off
  LShift : DSPBAPrim/LShift  primtype=lshift  nInputs=2  nOutputs=1  omode=Specify via dialog  otype=ufix(max_FFTStages)  scale=1  rndmethod=Unbiased  factor=1  satmethod=Symmetric  shift_vec=[0 1 2 -1]  value=0  inPortNames=['a'; 'b';]  outPortNames=[' ']  dspbaimage=dspba_prim.svg  text=fprintf('a << b');  style=Optimised  visibilities=8  version=20211007
  LShift1 : DSPBAPrim/LShift  primtype=lshift  nInputs=2  nOutputs=1  omode=Specify via dialog  otype=ufix(max_FFTStages)  scale=1  rndmethod=Unbiased  factor=1  satmethod=Symmetric  shift_vec=[0 1 2 -1]  value=0  inPortNames=['a'; 'b';]  outPortNames=[' ']  dspbaimage=dspba_prim.svg  text=fprintf('a << b');  style=Optimised  visibilities=8  version=20211007
  LShift2 : DSPBAPrim/LShift  primtype=lshift  nInputs=2  nOutputs=1  omode=Specify via dialog  otype=ufix(max_FFTStages+1)  scale=1  rndmethod=Unbiased  factor=1  satmethod=Symmetric  shift_vec=[0 1 2 -1]  value=0  inPortNames=['a'; 'b';]  outPortNames=[' ']  dspbaimage=dspba_prim.svg  text=fprintf('a << b');  style=Optimised  visibilities=8  version=20211007
  MemScope : Scope  NumInputPorts=5
  Not : DSPBAPrim/Not  primtype=not  nInputs=1  nOutputs=1  omode=Inherit via internal rule  otype=sfix(16)  scale=2^-15  rndmethod=Unbiased  factor=1  satmethod=Symmetric  shift_vec=[0 1 2 -1]  value=0  inPortNames=[' '; ' ';]  outPortNames=[' ']  dspbaimage=dspba_prim.svg  text=fprintf('~');  style=Optimised  visibilities=8  version=20211007
  Perm1 : DSPBAPrim/ChooseBits  primtype=choosebits  nInputs=1  nOutputs=1  omode=Inherit via internal rule  otype=fixdt(0,1,1)  scale=1  rndmethod=Unbiased  factor=1  satmethod=Symmetric  shift_vec=[0 1 2 -1]  value=[max_FFTStages-1 : -1 : 0]  inPortNames=[' '; ' ';]  outPortNames=[' ']  dspbaimage=dspba_prim.svg  text=fprintf('%s',dspba.perm2str(value));  style=Optimised  visibilities=1024  version=20211007
  Perm2 : DSPBAPrim/ChooseBits  primtype=choosebits  nInputs=1  nOutputs=1  omode=Inherit via internal rule  otype=fixdt(0,1,1)  scale=1  rndmethod=Unbiased  factor=1  satmethod=Symmetric  shift_vec=[0 1 2 -1]  value=[max_FFTStages-1 : -1 : 0]  inPortNames=[' '; ' ';]  outPortNames=[' ']  dspbaimage=dspba_prim.svg  text=fprintf('%s',dspba.perm2str(value));  style=Optimised  visibilities=1024  version=20211007
  RISING_EDGE : Subsystem
  ReadBankCounter : DSPBAPrim/Counter  primtype=counter  nInputs=1  nOutputs=1  omode=Specify via dialog  otype=ufix(1)  scale=1  rndmethod=Unbiased  factor=1  satmethod=Symmetric  shift_vec=[0 1 2 -1]  value=[0 2 1]  inPortNames=[' '; ' ';]  outPortNames=[' ']  dspbaimage=dspba_prim.svg  text=fprintf('counter\n[%d %d %d]', value(1), value(2), value(3));  style=Optimised  visibilities=8 + 1024  version=20211007
  ReadCounter : Subsystem
  Rising_edge : $bdroot/Rising_edge
  Rising_edge1 : $bdroot/Rising_edge
  Rising_edge2 : $bdroot/Rising_edge
  SRlatch : DSPBAControl/SRlatch
  SRlatch1 : DSPBAControl/SRlatch
  SampleDelay : DSPBAPrim/SampleDelay  primtype=sampdelay  nInputs=1  nOutputs=1  omode=Inherit via internal rule  otype=uint(16)  scale=2^-0  rndmethod=Unbiased  factor=1  satmethod=Symmetric  shift_vec=[0 1 2 -1]  floatPrecision=float32_m23  value=4  inPortNames=[' '; ' ';]  outPortNames=[' ']  dspbaimage=dspba_prim.svg  text=dpoly(1, eye(1,value+1), 'z')  style=Optimised  visibilities=8 + 1024  flexible=off  slackgroup=0  augmented=0  version=20211007  advOptions=[]
  Scope : Scope  NumInputPorts=6
  Select1 : DSPBAPrim/Select  primtype=select  nInputs=str2num(get_param(gcb,'value'))*2+1  nOutputs=1  omode=Inherit via internal rule  otype=sfix(16)  scale=2^-15  rndmethod=Unbiased  factor=1  satmethod=Symmetric  shift_vec=[0 1 2 -1]  value=1  inPortNames=['d'; '0'; 'a'; '1'; 'b'; '2'; 'c'; '3'; 'd'; '4'; 'e'; '5'; 'f'; '6'; 'g'; '7'; 'h'; '8'; 'i'; '9'; 'j']  outPortNames=[' ']  dspbaimage=dspba_prim_tall.svg  text=fprintf('%s', primtype);  style=Optimised  visibilities=8 + 1024  version=20211007
  StretchPulse : DSPBAControl/StretchPulse
  Sub1 : DSPBAPrim/Sub  primtype=sub  nInputs=2  nOutputs=1  omode=Specify via dialog  otype=ufix(ceil(log2(max_FFTStages)))  scale=1  rndmethod=Unbiased  factor=1  satmethod=Symmetric  shift_vec=[0 1 2 -1]  value=0  inPortNames=['+'; '-';]  outPortNames=[' ']  dspbaimage=dspba_prim.svg  text=fprintf('-');  style=Optimised  visibilities=8+2^17+2^18  floatRounding=correct  advOptions=[]  version=20211007
  Sub2 : DSPBAPrim/Sub  primtype=sub  nInputs=2  nOutputs=1  omode=Specify via dialog  otype=ufix(ceil(log2(max_FFTStages)))  scale=1  rndmethod=Unbiased  factor=1  satmethod=Symmetric  shift_vec=[0 1 2 -1]  value=0  inPortNames=['+'; '-';]  outPortNames=[' ']  dspbaimage=dspba_prim.svg  text=fprintf('-');  style=Optimised  visibilities=8+2^17+2^18  floatRounding=correct  advOptions=[]  version=20211007
  Terminator{,1..6} (7 alike) : Terminator
  WrCnt : Subsystem
  falling_edge : $bdroot/falling_edge
  falling_edge1 : $bdroot/falling_edge
  latch_0L{1..3,5} (4 alike) : DSPBAControl/latch_0L
  rdaddr : DSPBAPrim/BitCombine  primtype=bitcombine  nInputs=2  nOutputs=1  omode=Inherit via internal rule  otype=sfix(16)  scale=2^-15  rndmethod=Unbiased  factor=1  satmethod=Symmetric  shift_vec=[0 1 2 -1]  value=0  inPortNames=['l'; 'h';]  outPortNames=[' ']  dspbaimage=dspba_prim.svg  text=fprintf('[h,l]');  style=Optimised  visibilities=8+2  version=20211007
  ripple_comp : Subsystem
  wraddr : DSPBAPrim/BitCombine  primtype=bitcombine  nInputs=2  nOutputs=1  omode=Inherit via internal rule  otype=sfix(16)  scale=2^-15  rndmethod=Unbiased  factor=1  satmethod=Symmetric  shift_vec=[0 1 2 -1]  value=0  inPortNames=['l'; 'h';]  outPortNames=[' ']  dspbaimage=dspba_prim.svg  text=fprintf('[h,l]');  style=Optimised  visibilities=8+2  version=20211007
  qv : Outport
  q : Outport  Port=2
  g : Outport  Port=3
  ready : Outport  Port=4
  dout_rc_off : Outport  Port=5
  wires:
  d/1 -> Cplx2Vec2/1(cplx_in), DualMem1/1
  WrCnt/1(PhaseSel) -> BitExtract3/1
  WrCnt/2(WrAddr) -> LShift/1
  Not/1 -> rdaddr/2, CmpNE/2
  CmpNE/1 -> ready/1
  [NSubCarrs] -> latch_0L3/2
  BitExtract3/1 -> CmpNE/1, wraddr/2
  BitExtract5/1 -> Perm2/1
  Perm2/1 -> ripple_comp/4(addr_in), rdaddr/1
  LShift/1 -> wraddr/1
  Const/1 -> Sub1/1
  [FFTSize] -> Sub1/2
  Sub1/1 -> LShift/2
  wraddr/1 -> MemScope/2, DualMem1/2
  rdaddr/1 -> MemScope/4, DualMem1/4
  ReadBankCounter/1 -> Not/1
  DualMem1/1 -> Terminator/1
  ReadCounter/1(count) -> LShift1/1, BitExtract5/1
  Const1/1 -> Select1/1
  ripple_comp/1(dout) -> Cplx2Vec1/1(cplx_in), Select1/3
  latch_0L2/1 -> StretchPulse/2, ReadCounter/2(fft_size)
  Const2/1 -> Sub2/1
  BitExtract1/1 -> Perm1/1
  LShift1/1 -> BitExtract1/1
  Perm1/1 -> CheckLegalRange/1(addr_in)
  CheckLegalRange/1(addr_legal) -> Select1/2
  Cplx2Vec2/1(vec_out) -> MemScope/1
  Cplx2Vec1/1(vec_out) -> MemScope/5
  [FFTSize] -> latch_0L1/2, LShift2/2
  Const4/1 -> LShift2/1
  LShift2/1 -> FIFO/2
  Sub2/1 -> LShift1/2
  Rising_edge2/1 -> ReadBankCounter/1
  v/1 -> Rising_edge/1, falling_edge/1, g/1, MemScope/3, DualMem1/3, WrCnt/1(vin)  "go"
  FIFO/3 -> Terminator2/1
  FIFO/4 -> Terminator3/1
  FIFO/1 -> Terminator1/1
  Rising_edge/1 -> FIFO/1, FIFO1/1, Scope/4
  RISING_EDGE/1(q) -> StretchPulse/1, SRlatch1/2, SRlatch/2, FIFO/3, latch_0L2/1, latch_0L3/1, latch_0L1/1
  ReadCounter/2(read_done) -> Rising_edge2/1, Rising_edge1/1  "go"
  And/1 -> RISING_EDGE/1(d)
  FIFO/2 -> latch_0L2/2
  SRlatch/1 -> And/1
  SRlatch1/1 -> And/2
  falling_edge/1 -> SRlatch/1
  latch_0L1/1 -> Sub2/2, CheckLegalRange/2(fftsizein)
  latch_0L3/1 -> CheckLegalRange/3(nsc)
  FIFO1/1 -> Terminator4/1
  FIFO1/3 -> Terminator5/1
  FIFO1/4 -> Terminator6/1
  [chan] -> Scope/5, FIFO1/2
  FIFO1/2 -> Scope/2, latch_0L5/2
  latch_0L5/1 -> Scope/3, ReadCounter/3(chn)
  Rising_edge1/1 -> SRlatch1/1
  StretchPulse/1 -> falling_edge1/1, qv/1, ReadCounter/1(enable)
  SampleDelay/1 -> Scope/1, latch_0L5/1, Scope/6, FIFO1/3
  DC_SC_EN/1 -> CheckLegalRange/4(DC_SC_EN), WrCnt/2(DC_SC_EN)
  falling_edge1/1 -> SampleDelay/1
  Select1/1 -> q/1
  DualMem1/2 -> ripple_comp/2(din)
  ripple_comp_en/1 -> ripple_comp/1(ripple_comp_en)
  rc_bw_sel/1 -> ripple_comp/3(rc_bw_sel)
  ripple_comp/2(dout_rc_off) -> dout_rc_off/1

== system lib_lowphy/FFT_S2B/CPRemoval/Mem_rd_sub1/Incr_Symbol_out_val/Sym_counter_meta_data/Rising edge1 ==
  d : Inport
  And : DSPBAPrim/And  primtype=and  nInputs=2  nOutputs=1  omode=Inherit via internal rule  otype=sfix(16)  scale=2^-15  rndmethod=Unbiased  factor=1  satmethod=Symmetric  shift_vec=[0 1 2 -1]  value=0  inPortNames=[' '; ' '; ' '; ' '; ' '; ' '; ' '; ' '; ' '; ' '; ' '; ' '; ' '; ' '; ' '; ' '; ]  outPortNames=[' ']  dspbaimage=dspba_prim.svg  text=fprintf('&');  style=Optimised  visibilities=8+2  version=20211007
  Not1 : DSPBAPrim/Not  primtype=not  nInputs=1  nOutputs=1  omode=Inherit via internal rule  otype=sfix(16)  scale=2^-15  rndmethod=Unbiased  factor=1  satmethod=Symmetric  shift_vec=[0 1 2 -1]  value=0  inPortNames=[' '; ' ';]  outPortNames=[' ']  dspbaimage=dspba_prim.svg  text=fprintf('~');  style=Optimised  visibilities=8  version=20211007
  SampleDelay : DSPBAPrim/SampleDelay  primtype=sampdelay  nInputs=1  nOutputs=1  omode=Inherit via internal rule  otype=sfix(16)  scale=2^-15  rndmethod=Unbiased  factor=1  satmethod=Symmetric  shift_vec=[0 1 2 -1]  floatPrecision=float32_m23  value=1  inPortNames=[' '; ' ';]  outPortNames=[' ']  dspbaimage=dspba_prim.svg  text=dpoly(1, eye(1,value+1), 'z')  style=Optimised  visibilities=8 + 1024 + 2^17 + 2^18  flexible=off  slackgroup=0  augmented=0  version=20211007  advOptions=[]
  q : Outport
  wires:
  Not1/1 -> And/1
  d/1 -> And/2, SampleDelay/1
  SampleDelay/1 -> Not1/1
  And/1 -> q/1

== system lib_lowphy/FFT_S2B/CPRemoval/Mem_rd_sub1/Incr_Symbol_out_val/Sym_counter_meta_data/Subsystem ==
  cntr : Inport
  And : DSPBAPrim/And  primtype=and  nInputs=2  nOutputs=1  omode=Inherit via internal rule  otype=sfix(16)  scale=2^-15  rndmethod=Unbiased  factor=1  satmethod=Symmetric  shift_vec=[0 1 2 -1]  value=0  inPortNames=[' '; ' '; ' '; ' '; ' '; ' '; ' '; ' '; ' '; ' '; ' '; ' '; ' '; ' '; ' '; ' '; ]  outPortNames=[' ']  dspbaimage=dspba_prim.svg  text=fprintf('&');  style=Optimised  visibilities=8+2  version=20211007
  CmpEQ1 : DSPBAPrim/CmpEQ  primtype=cmpeq  nInputs=2  nOutputs=1  omode=boolean  otype=sfix(16)  scale=2^-15  rndmethod=Unbiased  factor=1  satmethod=Symmetric  shift_vec=[0 1 2 -1]  value=0  inPortNames=[' '; ' ';]  outPortNames=[' ']  dspbaimage=dspba_prim.svg  text=fprintf('==');  style=Optimised  visibilities=0  advOptions=[]  version=20211007
  CmpEQ3 : DSPBAPrim/CmpEQ  primtype=cmpeq  nInputs=2  nOutputs=1  omode=boolean  otype=sfix(16)  scale=2^-15  rndmethod=Unbiased  factor=1  satmethod=Symmetric  shift_vec=[0 1 2 -1]  value=0  inPortNames=[' '; ' ';]  outPortNames=[' ']  dspbaimage=dspba_prim.svg  text=fprintf('==');  style=Optimised  visibilities=0  advOptions=[]  version=20211007
  Const13 : DSPBAPrim/Const  primtype=const  nInputs=0  nOutputs=1  omode=Inherit via internal rule  otype=sfix(16)  scale=2^-15  rndmethod=Unbiased  factor=1  satmethod=Symmetric  shift_vec=[0 1 2 -1]  value=13  inPortNames=['+'; '+';]  outPortNames=[' ']  dspbaimage=dspba_prim.svg  text=fprintf('%s', num2str(value));  style=Optimised  visibilities=8 + 1024  floatPrecision=float32_m23  warnSaturation=on  version=20211007  SampleTime=inf
  Const5 : DSPBAPrim/Const  primtype=const  nInputs=0  nOutputs=1  omode=Inherit via internal rule  otype=sfix(16)  scale=2^-15  rndmethod=Unbiased  factor=1  satmethod=Symmetric  shift_vec=[0 1 2 -1]  value=0  inPortNames=['+'; '+';]  outPortNames=[' ']  dspbaimage=dspba_prim.svg  text=fprintf('%s', num2str(value));  style=Optimised  visibilities=8 + 1024  floatPrecision=float32_m23  warnSaturation=on  version=20211007  SampleTime=inf
  SampleDelay2 : DSPBAPrim/SampleDelay  primtype=sampdelay  nInputs=1  nOutputs=1  omode=Inherit via internal rule  otype=sfix(16)  scale=2^-15  rndmethod=Unbiased  factor=1  satmethod=Symmetric  shift_vec=[0 1 2 -1]  floatPrecision=float32_m23  value=1  inPortNames=[' '; ' ';]  outPortNames=[' ']  dspbaimage=dspba_prim.svg  text=dpoly(1, eye(1,value+1), 'z')  style=Optimised  visibilities=8 + 1024 + 2^17 + 2^18  flexible=off  slackgroup=0  augmented=0  version=20211007  advOptions=[]
  sym1_det : Outport
  wires:
  Const13/1 -> CmpEQ3/2
  And/1 -> sym1_det/1
  SampleDelay2/1 -> And/2
  CmpEQ3/1 -> SampleDelay2/1
  cntr/1 -> CmpEQ1/1, CmpEQ3/1
  CmpEQ1/1 -> And/1
  Const5/1 -> CmpEQ1/2

== system lib_lowphy/FFT_S2B/SignalProcessing/BRandSCSelect1/Transpose/ReadCounter/Address Comparison ==
  rd_addr : Inport
  nsc : Inport  Port=2
  CmpEQ1 : DSPBAPrim/CmpEQ  primtype=cmpeq  nInputs=2  nOutputs=1  omode=boolean  otype=sfix(16)  scale=2^-15  rndmethod=Unbiased  factor=1  satmethod=Symmetric  shift_vec=[0 1 2 -1]  value=0  inPortNames=[' '; ' ';]  outPortNames=[' ']  dspbaimage=dspba_prim.svg  text=fprintf('==');  style=Optimised  visibilities=0  advOptions=[]  version=20211007
  CmpEQ2 : DSPBAPrim/CmpEQ  primtype=cmpeq  nInputs=2  nOutputs=1  omode=boolean  otype=sfix(16)  scale=2^-15  rndmethod=Unbiased  factor=1  satmethod=Symmetric  shift_vec=[0 1 2 -1]  value=0  inPortNames=[' '; ' ';]  outPortNames=[' ']  dspbaimage=dspba_prim.svg  text=fprintf('==');  style=Optimised  visibilities=0  advOptions=[]  version=20211007
  Const6 : DSPBAPrim/Const  primtype=const  nInputs=0  nOutputs=1  omode=Specify via dialog  otype=ufix(ceil(log2(max_NSubcarriers)))  scale=1  rndmethod=Unbiased  factor=1  satmethod=Symmetric  shift_vec=[0 1 2 -1]  value=0  inPortNames=['+'; '+';]  outPortNames=[' ']  dspbaimage=dspba_prim.svg  text=fprintf('%s', num2str(value));  style=Optimised  visibilities=8 + 1024  floatPrecision=float32_m23  warnSaturation=on  version=20211007  SampleTime=inf
  Or1 : DSPBAPrim/Or  primtype=or  nInputs=2  nOutputs=1  omode=Inherit via internal rule  otype=sfix(16)  scale=2^-15  rndmethod=Unbiased  factor=1  satmethod=Symmetric  shift_vec=[0 1 2 -1]  value=0  inPortNames=[' '; ' '; ' '; ' '; ' '; ' '; ' '; ' '; ' '; ' '; ' '; ' '; ' '; ' '; ' '; ' '; ]  outPortNames=[' ']  dspbaimage=dspba_prim.svg  text=fprintf('|');  style=Optimised  visibilities=8+2  version=20211007
  rd_done : Outport
  wires:
  CmpEQ1/1 -> Or1/2  "go"
  CmpEQ2/1 -> Or1/1  "go"
  rd_addr/1 -> CmpEQ1/1, CmpEQ2/1
  Const6/1 -> CmpEQ1/2
  nsc/1 -> CmpEQ2/2
  Or1/1 -> rd_done/1

== system lib_lowphy/FFT_S2B/SignalProcessing/BRandSCSelect1/Transpose/ReadCounter/RISING_EDGE ==
  d : Inport
  And : DSPBAPrim/And  primtype=and  nInputs=2  nOutputs=1  omode=Inherit via internal rule  otype=sfix(16)  scale=2^-15  rndmethod=Unbiased  factor=1  satmethod=Symmetric  shift_vec=[0 1 2 -1]  value=0  inPortNames=[' '; ' '; ' '; ' '; ' '; ' '; ' '; ' '; ' '; ' '; ' '; ' '; ' '; ' '; ' '; ' '; ]  outPortNames=[' ']  dspbaimage=dspba_prim.svg  text=fprintf('&');  style=Optimised  visibilities=8+2  version=20211007
  Not1 : DSPBAPrim/Not  primtype=not  nInputs=1  nOutputs=1  omode=Inherit via internal rule  otype=sfix(16)  scale=2^-15  rndmethod=Unbiased  factor=1  satmethod=Symmetric  shift_vec=[0 1 2 -1]  value=0  inPortNames=[' '; ' ';]  outPortNames=[' ']  dspbaimage=dspba_prim.svg  text=fprintf('~');  style=Optimised  visibilities=8  version=20211007
  SampleDelay : DSPBAPrim/SampleDelay  primtype=sampdelay  nInputs=1  nOutputs=1  omode=Inherit via internal rule  otype=sfix(16)  scale=2^-15  rndmethod=Unbiased  factor=1  satmethod=Symmetric  shift_vec=[0 1 2 -1]  floatPrecision=float32_m23  value=1  inPortNames=[' '; ' ';]  outPortNames=[' ']  dspbaimage=dspba_prim.svg  text=dpoly(1, eye(1,value+1), 'z')  style=Optimised  visibilities=8 + 1024 + 2^17 + 2^18  flexible=off  slackgroup=0  augmented=0  version=20211007  advOptions=[]
  q : Outport
  wires:
  And/1 -> q/1
  Not1/1 -> And/1
  d/1 -> SampleDelay/1, And/2
  SampleDelay/1 -> Not1/1

== system lib_lowphy/FFT_S2B/SignalProcessing/BRandSCSelect1/Transpose/SampleCounter/RISING_EDGE ==
  d : Inport
  And : DSPBAPrim/And  primtype=and  nInputs=2  nOutputs=1  omode=Inherit via internal rule  otype=sfix(16)  scale=2^-15  rndmethod=Unbiased  factor=1  satmethod=Symmetric  shift_vec=[0 1 2 -1]  value=0  inPortNames=[' '; ' '; ' '; ' '; ' '; ' '; ' '; ' '; ' '; ' '; ' '; ' '; ' '; ' '; ' '; ' '; ]  outPortNames=[' ']  dspbaimage=dspba_prim.svg  text=fprintf('&');  style=Optimised  visibilities=8+2  version=20211007
  Not1 : DSPBAPrim/Not  primtype=not  nInputs=1  nOutputs=1  omode=Inherit via internal rule  otype=sfix(16)  scale=2^-15  rndmethod=Unbiased  factor=1  satmethod=Symmetric  shift_vec=[0 1 2 -1]  value=0  inPortNames=[' '; ' ';]  outPortNames=[' ']  dspbaimage=dspba_prim.svg  text=fprintf('~');  style=Optimised  visibilities=8  version=20211007
  SampleDelay : DSPBAPrim/SampleDelay  primtype=sampdelay  nInputs=1  nOutputs=1  omode=Inherit via internal rule  otype=sfix(16)  scale=2^-15  rndmethod=Unbiased  factor=1  satmethod=Symmetric  shift_vec=[0 1 2 -1]  floatPrecision=float32_m23  value=1  inPortNames=[' '; ' ';]  outPortNames=[' ']  dspbaimage=dspba_prim.svg  text=dpoly(1, eye(1,value+1), 'z')  style=Optimised  visibilities=8 + 1024 + 2^17 + 2^18  flexible=off  slackgroup=0  augmented=0  version=20211007  advOptions=[]
  q : Outport
  wires:
  And/1 -> q/1
  Not1/1 -> And/1
  d/1 -> SampleDelay/1, And/2
  SampleDelay/1 -> Not1/1

== system lib_lowphy/iFFT_B2S/B2S/B2S_Inst/CB/Rdaddr_gen1/rd_addr_1024 ==
  sampleaddr_reg : Inport
  cpin : Inport  Port=2
  Add2 : DSPBAPrim/Add  primtype=add  nInputs=evalAionMaskParam(gcb,'value',1)  nOutputs=1  omode=Inherit via internal rule with word growth  otype=fixdt(0,12,0)  scale=0  rndmethod=Unbiased  factor=1  satmethod=Symmetric  shift_vec=[0 1 2 -1]  value=2  inPortNames=[' '; ' ';]  outPortNames=[' ']  dspbaimage=dspba_prim.svg  text=fprintf('+');  style=Optimised  visibilities=1032+2^17+2^18+2^19  genFPC=off  floatRounding=correct  advOptions=[]  version=20211007
  BitCombine2 : DSPBAPrim/BitCombine  primtype=bitcombine  nInputs=2  nOutputs=1  omode=Inherit via internal rule  otype=sfix(16)  scale=2^-15  rndmethod=Unbiased  factor=1  satmethod=Symmetric  shift_vec=[0 1 2 -1]  value=0  inPortNames=['l'; 'h';]  outPortNames=[' ']  dspbaimage=dspba_prim.svg  text=fprintf('[h,l]');  style=Optimised  visibilities=8+2  version=20211007
  ChooseBits : DSPBAPrim/ChooseBits  primtype=choosebits  nInputs=1  nOutputs=1  omode=Inherit via internal rule  otype=fixdt(0,1,1)  scale=1  rndmethod=Unbiased  factor=1  satmethod=Symmetric  shift_vec=[0 1 2 -1]  value=[0,1]  inPortNames=[' '; ' ';]  outPortNames=[' ']  dspbaimage=dspba_prim.svg  text=fprintf('%s',dspba.perm2str(value));  style=Optimised  visibilities=1024  version=20211007
  Constant1 : Constant  Value=0  OutDataTypeStr=fixdt(0,2,0)
  Constant7 : Constant  Value=1024  OutDataTypeStr=fixdt(0,15,0)
  Constant8 : Constant  Value=2  OutDataTypeStr=fixdt(0,15,0)
  Convert : DSPBAPrim/Convert  primtype=convert  nInputs=1  nOutputs=1  omode=Specify via dialog  otype=fixdt(0,10,0)  scale=0  rndmethod=Biased  factor=1  satmethod=None  shift_vec=[0 1 2 -1]  value=round([0:255]/17)  inPortNames=[' '; ' ';]  outPortNames=[' '; 'c']  dspbaimage=dspba_prim_wide.svg  text=fprintf('convert');  style=Optimised  visibilities=8+64+256+2^17  clipdetect=off  floatPrecision=float32_m23  advOptions=[]  version=20211007
  Shift : DSPBAPrim/Shift  primtype=shift  nInputs=2  nOutputs=1  omode=Specify via dialog  otype=fixdt(0,12,0)  scale=0  rndmethod=Unbiased  factor=1  satmethod=Symmetric  shift_vec=[0 1 2 -1]  value=0  inPortNames=['a'; 'b';]  outPortNames=[' ']  dspbaimage=dspba_prim.svg  text=fprintf('a >> b');  style=Optimised  visibilities=8  version=20211007
  Sub : DSPBAPrim/Sub  primtype=sub  nInputs=2  nOutputs=1  omode=Specify via dialog  otype=fixdt(0,13,0)  scale=0  rndmethod=Unbiased  factor=1  satmethod=Symmetric  shift_vec=[0 1 2 -1]  value=0  inPortNames=['+'; '-';]  outPortNames=[' ']  dspbaimage=dspba_prim.svg  text=fprintf('-');  style=Optimised  visibilities=8+2^17+2^18  floatRounding=correct  advOptions=[]  version=20211007
  AntNo : Outport
  rdaddr1 : Outport  Port=2  OutDataTypeStr=fixdt(0,12,0)
  wires:
  cpin/1 -> Sub/2
  Shift/1 -> Add2/2
  sampleaddr_reg/1 -> Shift/1, ChooseBits/1
  Constant8/1 -> Shift/2
  Constant7/1 -> Sub/1
  ChooseBits/1 -> AntNo/1
  Sub/1 -> Add2/1
  Add2/1 -> Convert/1
  Convert/1 -> BitCombine2/1
  BitCombine2/1 -> rdaddr1/1
  Constant1/1 -> BitCombine2/2
